simulink model "R7014E_Pumpcurve"  (R2016b)
settings: Solver=ode5  StartTime=0.0  StopTime=inf  RelTol=1e-3  EnableMultiTasking=on
undefined symbols (not defined in the file): National_Instruments, PCI
libraries: rtwinlib x2
settings Model: Creator=wolfgang  LastModifiedBy=wolfgang
settings Model: ModifiedHistory=|
  | Created an adjusted empty Simulink diagram for the lab assignments
  | in the course R0002E
settings DataIOCC: SaveFormat=Array  SignalLoggingSaveFormat=ModelDataLogs  SaveOutput=off  SignalLogging=off  DSMLogging=off  SaveTime=off
settings OptimizationCC: ExpressionDepthLimit=2147483647  LifeSpan=inf
settings DebuggingCC: UnderspecifiedInitializationDetection=Classic  MergeDetectMultiDrivingBlocksExec=none  SolverPrmCheckMsg=warning  FcnCallInpInsideContextMsg=warning  StateNameClashWarn=warning  SFUnexpectedBacktrackingDiag=warning  SFNoUnconditionalDefaultTransitionDiag=warning  SFExecutionAtInitializationDiag=none
settings HardwareCC: ProdBitPerPointer=32  ProdBitPerSizeT=32  ProdBitPerPtrDiffT=32  ProdLargestAtomicFloat=None  ProdIntDivRoundTo=Undefined  ProdEndianess=Unspecified  ProdWordSize=32  ProdHWDeviceType=32-bit Generic
settings ModelReferenceCC: PropagateSignalLabelsOutOfModel=off
settings GRTTargetCC: TargetLangStandard=C89/C90 (ANSI)  GeneratePreprocessorConditionals=Disable all
settings ConfigComp: CovMetricSettings=dw  CovHtmlReporting=on  CovSaveCumulativeToWorkspaceVar=on  CovSaveSingleToWorkspaceVar=on  CovExternalEMLEnable=off  CovSFcnEnable=off

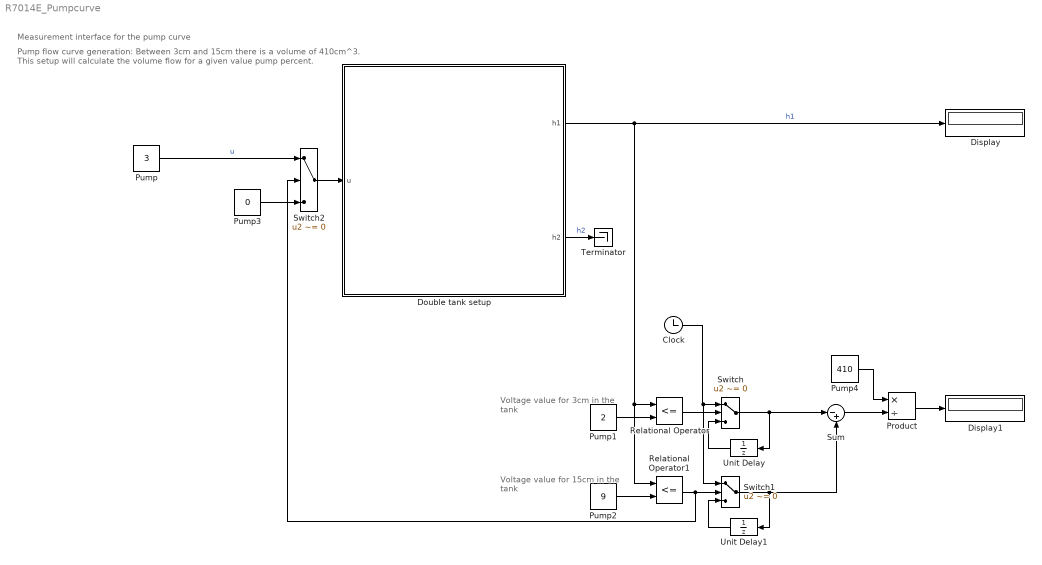
== system R7014E_Pumpcurve ==
  note: Voltage value for
      | 3cm in the tank
  note: Measurement interface for the pump curve
  note: Pump flow curve generation:
      | Between 3cm and 15cm there is a volume of
      | 410cm^3. This setup will calculate the
      | volume flow for a given value pump percent.
  note: Voltage value for
      | 15cm in the tank
  Clock : Clock
  Display : Display
  Display1 : Display
  Double tank setup : Subsystem  AncestorBlock=R0002E_lib/Double tank setup  StopFcn=|  mask(Realtime interface for the tank process){ts=0.02, h1_ch=0, h2_ch=1, u_ch=0}
      | chn =get_param(gcb,'u_ch');                          
      | s = daq.createSession('ni');                         
      | channel = ['ao',chn];                                
      | s.addAnalogOutputChannel('Dev1', channel, 'Voltage');
      | x = zeros(5,1);                                      
      | s.queueOutputData(x);                                
      | lh = s.addlistener('DataRequired', ...               
      | @(src,event) src.queueOutputData(x));                
      | s.startBackground();                                 
      | s.wait();                                            
      | s.stop();                                            
      | delete(lh);                                          
      | clear chn;                                           
      | clear s;                                             
      | clear channel;                                       
      | clear lh;                                            
      | clear x;
      mask prompts: ts "Sample time"; h1_ch "A/D Channel for upper tank"; h2_ch "A/D Channel for lower tank"; u_ch "D/A Channel for pump"
      mask help:
      | This block represents the physical interface from the computer to the tank process.
      |
      | The input u is the voltage that is provided for the pump, the output h1 is the measured level in the upper tank in [V] and the output h2 is the
      | measured level in the lower tank in [V].
      |
      | You need to provide the sample rate at which the voltage to the pump is updated and the level measurements are sampled. The sample rate should not be less than 0.02 seconds.
      mask Display:
      | x=363;
      | y=381;
      | image(imread('tank_icon.jpg'));
      | text(250/x,309/y,'Sensor');
      | text(260/x,169/y,'Sensor');
      | text(335/x,289/y,'A');
      | text(351/x,283/y,'D');
      | text(335/x,100/y,'A');
      | text(351/x,95/y,'D');
      | text(22/x,187/y,'A');
      | text(5/x,195/y,'D');
      | text(225/x,278/y,'h_1','texmode','on');
      | text(225/x,146/y,'h_2','texmode','on');
      | text(300/x,270/y,sprintf('AI-%d',h1_ch));
      | text(300/x,80/y,sprintf('AI-%d',h2_ch));
      | text(40/x,173/y,sprintf('AO-%d',u_ch));
  Product : Product  Inputs=*/
  Pump : Constant  Value=3
  Pump1 : Constant  Value=2
  Pump2 : Constant  Value=9
  Pump3 : Constant  Value=0
  Pump4 : Constant  Value=410
  Relational Operator : RelationalOperator  Operator=<=  OutDataTypeStr=boolean  RndMeth=Nearest
  Relational Operator1 : RelationalOperator  Operator=<=  OutDataTypeStr=boolean  RndMeth=Nearest
  Sum : Sum  Inputs=|-+
  Switch : Switch  Criteria=u2 ~= 0
  Switch1 : Switch  Criteria=u2 ~= 0
  Switch2 : Switch  Criteria=u2 ~= 0
  Terminator : Terminator
  Unit Delay : UnitDelay  SampleTime=-1
  Unit Delay1 : UnitDelay  SampleTime=-1
  wires:
  Double tank setup/1(h1) -> Relational Operator1/1, Relational Operator/1, Display/1  "h1"
  Double tank setup/2(h2) -> Terminator/1  "h2"
  Pump1/1 -> Relational Operator/2
  Switch/1 -> Sum/1, Unit Delay/1
  Unit Delay/1 -> Switch/3
  Clock/1 -> Switch1/1, Switch/1
  Relational Operator/1 -> Switch/2
  Pump2/1 -> Relational Operator1/2
  Switch1/1 -> Sum/2, Unit Delay1/1
  Unit Delay1/1 -> Switch1/3
  Relational Operator1/1 -> Switch2/2, Switch1/2
  Sum/1 -> Product/2
  Pump4/1 -> Product/1
  Product/1 -> Display1/1
  Pump/1 -> Switch2/1  "u"
  Switch2/1 -> Double tank setup/1(u)
  Pump3/1 -> Switch2/3

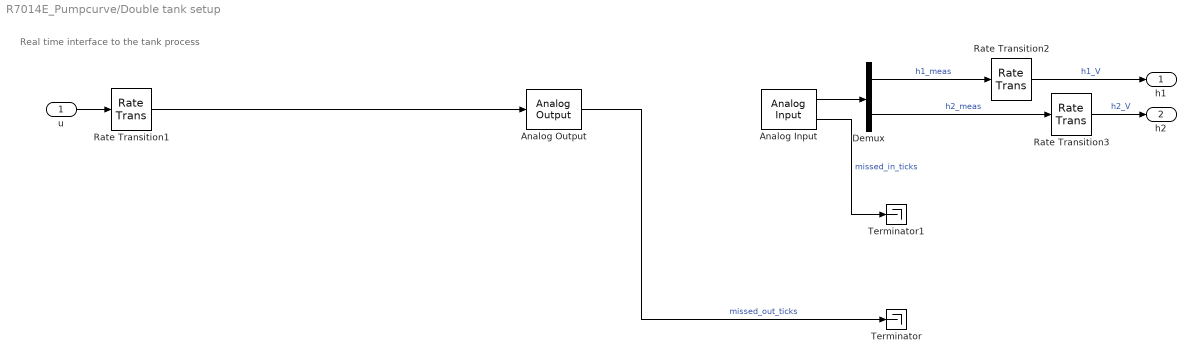
== system R7014E_Pumpcurve/Double tank setup ==
  note: Real time interface to the tank process
  u : Inport
  Analog Input : rtwinlib/Analog Input  SampleTime=ts  MaxMissedTicks=500000000  ShowMissedTicks=on  YieldWhenWaiting=off  DrvName=National_Instruments/PCI-6024E  DrvAddress=4294967295  DrvOptions=[0 0 0 0 0 0]  Channels=[h1_ch+1,h2_ch+1]  RangeMode=1  VoltRange=1  DataType=1
      settings: AttributesFormatString=National Instruments\nPCI-6024E [auto]
  Analog Output : rtwinlib/Analog Output  SampleTime=ts  MaxMissedTicks=500000000  ShowMissedTicks=on  YieldWhenWaiting=off  DrvName=National_Instruments/PCI-6024E  DrvAddress=4294967295  DrvOptions=[0 0 0 0 0 0]  Channels=u_ch+1  RangeMode=1  VoltRange=1  InitialValue=0  FinalValue=0
      settings: AttributesFormatString=National Instruments\nPCI-6024E [auto]
  Demux : Demux  Outputs=2
  Rate Transition1 : RateTransition  OutPortSampleTime=ts
  Rate Transition2 : RateTransition
  Rate Transition3 : RateTransition
  Terminator : Terminator
  Terminator1 : Terminator
  h1 : Outport
  h2 : Outport  Port=2
  wires:
  Rate Transition1/1 -> Analog Output/1
  Rate Transition3/1 -> h2/1  "h2_V"
  Rate Transition2/1 -> h1/1  "h1_V"
  Analog Input/2 -> Terminator1/1  "missed_in_ticks"
  Demux/2 -> Rate Transition3/1  "h2_meas"
  Demux/1 -> Rate Transition2/1  "h1_meas"
  Analog Input/1 -> Demux/1
  Analog Output/1 -> Terminator/1  "missed_out_ticks"
  u/1 -> Rate Transition1/1
